simulink model "SST_v2_21b"  (R2021b)
settings: Solver=ode1be  StartTime=0.0  StopTime=1  FixedStep=Ts  RelTol=1e-3
values from neighbouring files (symbols this model uses):
  Kiv = 1/Tpv    (= 22527.3933103)    [DC_Grid_Light.m]
  Kpv = Tzv/Tpv    (= 0.187728277586)    [DC_Grid_Light.m]
undefined symbols (not defined in the file or in its folder): Cout, Imax, Kii, Kpi, Lfilter, Lgrid, Rfilter, Rgrid, RLoad, Ts, VAC_pk
libraries: simulink x62, spsVoltageMeasurementLib x21, spsParallelRLCBranchLib x15, spsFullBridgeConverterLib x15, spsACVoltageSourceLib x3, spsCurrentMeasurementLib x3, spsGroundLib x3, slpidlib x3, spsSeriesRLCBranchLib x3, spspowerguiLib x1
(part 1 of 2)
settings Model: Creator=velo  LastModifiedBy=MiguelVelo
settings DataIOCC: InitialState=out1.xFinal  SaveOperatingPoint=on
settings DebuggingCC: UnconnectedInputMsg=none  UnconnectedOutputMsg=none  UnconnectedLineMsg=none
settings ModelReferenceCC: EnableRefExpFcnMdlSchedulingChecks=off
settings RTWCC: GPUComputeCapability=5.0  DLArmComputeVersion=20.02.1

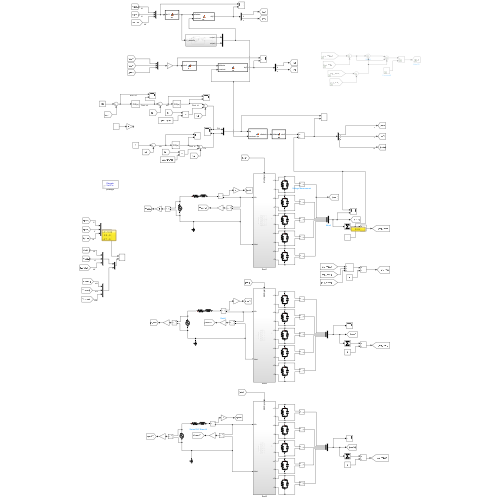
[thumbnail: Simulink's stored preview of the top-level diagram]
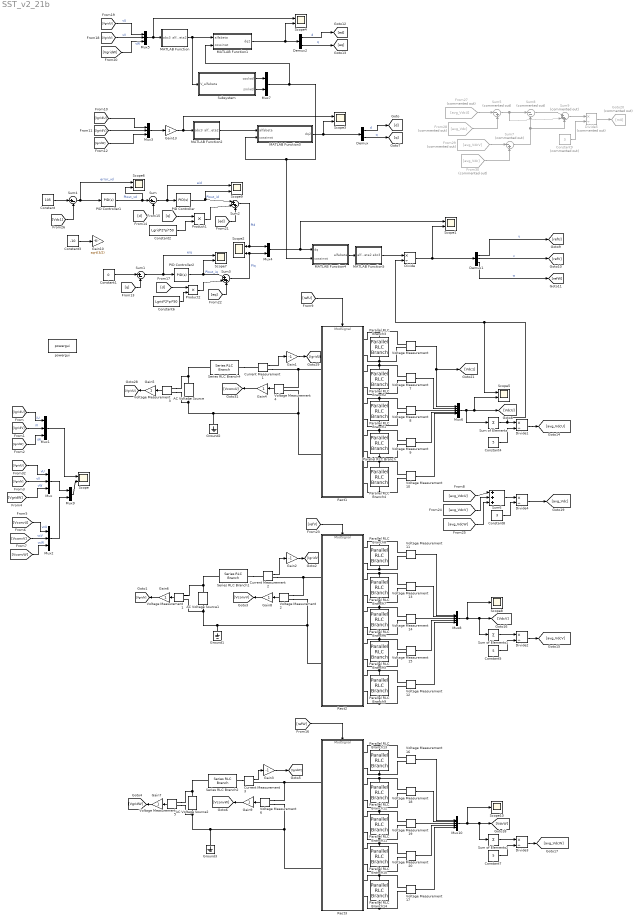
== system SST_v2_21b ==
  AC Voltage Source : spsACVoltageSourceLib/AC Voltage Source  Amplitude=VAC_pk  Phase=0  Frequency=50  SampleTime=0  Measurements=None  BusType=swing  Pref=10e3  Qref=0  Qmin=-inf  Qmax=+inf
  AC Voltage Source1 : spsACVoltageSourceLib/AC Voltage Source  Amplitude=VAC_pk  Phase=-120  Frequency=50  SampleTime=0  Measurements=None  BusType=swing  Pref=10e3  Qref=0  Qmin=-inf  Qmax=+inf
  AC Voltage Source2 : spsACVoltageSourceLib/AC Voltage Source  Amplitude=VAC_pk  Phase=120  Frequency=50  SampleTime=0  Measurements=None  BusType=swing  Pref=10e3  Qref=0  Qmin=-inf  Qmax=+inf
  Constant : Constant  Value=105
  Constant1 : Constant  Value=0
  Constant2 : Constant  Value=Lgrid*2*pi*50
  Constant3 : Constant  Value=-10
  Constant4 : Constant  Value=5
  Constant5 : Constant  Value=5
  Constant6 : Constant  Value=Lgrid*2*pi*50
  Constant7 : Constant  Value=5
  Constant8 : Constant  Value=3
  Constant9 : Constant  Commented=on  Value=3
  Current Measurement1 : spsCurrentMeasurementLib/Current Measurement  PhasorSimulation=off  OutputType=Complex  PSBequivalent=0
  Current Measurement2 : spsCurrentMeasurementLib/Current Measurement  PhasorSimulation=off  OutputType=Complex  PSBequivalent=0
  Current Measurement3 : spsCurrentMeasurementLib/Current Measurement  PhasorSimulation=off  OutputType=Complex  PSBequivalent=0
  Demux : Demux  Outputs=2
  Demux1 : Demux  Outputs=3
  Demux2 : Demux  Outputs=2
  Divide{,1..4} (5 alike) : Product  Inputs=*/
  Divide5 : Product  Commented=on  Inputs=*/
  From27 : From  Commented=on  GotoTag=avg_VdcU
  From28 : From  Commented=on  GotoTag=avg_Vdc
  From29 : From  Commented=on  GotoTag=avg_VdcV
  From30 : From  Commented=on  GotoTag=avg_Vdc
  Gain1 : Gain  Gain=-1
  Gain10 : Gain  Gain=sqrt(3/2)
  Gain{4..9,13} (7 alike) : Gain
  Gain2 : Gain  Gain=-1
  Gain3 : Gain  Gain=-1
  Goto20 : Goto  Commented=on  GotoTag=m0
  Ground1 : spsGroundLib/Ground  LConnTagsString=a
  Ground2 : spsGroundLib/Ground  LConnTagsString=a
  Ground3 : spsGroundLib/Ground  LConnTagsString=a
  MATLAB Function : MATLAB Function  TreatAsAtomicUnit=on
  MATLAB Function1 : MATLAB Function  TreatAsAtomicUnit=on
  MATLAB Function2 : MATLAB Function  TreatAsAtomicUnit=on
  MATLAB Function3 : MATLAB Function  TreatAsAtomicUnit=on
  MATLAB Function4 : MATLAB Function  TreatAsAtomicUnit=on
  MATLAB Function5 : MATLAB Function  TreatAsAtomicUnit=on
  Mux{,1..3,5} (5 alike) : Mux  Inputs=3
  Mux10 : Mux  Inputs=5
  Mux4 : Mux  Inputs=2
  Mux6 : Mux  Inputs=5
  Mux7 : Mux  Inputs=2
  Mux8 : Mux  Inputs=5
  Mux9 : Mux  Inputs=2
  PID Controller : slpidlib/PID Controller  Controller=PID  Form=Parallel  TimeDomain=Continuous-time  UseExternalTs=off  SampleTime=-1  IntegratorMethod=Forward Euler  FilterMethod=Forward Euler  ControllerParametersSource=internal  P=Kpi  I=Kii  D=0  UseFilter=on  N=100  TunerSelectOption=Transfer Function Based (PID Tuner App)  InitialConditionSource=internal  InitialConditionForIntegrator=0  InitialConditionForFilter=0  DifferentiatorICPrevScaledInput=0  ExternalReset=none  TrackingMode=off  Kt=1  LimitOutput=off  SatLimitsSource=internal  UpperSaturationLimit=Imax  LowerSaturationLimit=-Imax  LinearizeAsGain=on  AntiWindupMode=clamping  Kb=1  POutMin=[]  POutMax=[]  IOutMin=[]  IOutMax=[]  DOutMin=[]  DOutMax=[]  NOutMin=[]  NOutMax=[]  SumOutMin=[]  SumOutMax=[]  SaturationOutMin=[]  SaturationOutMax=[]  PParamMin=[]  PParamMax=[]  IParamMin=[]  IParamMax=[]  DParamMin=[]  DParamMax=[]  NParamMin=[]  NParamMax=[]  KbParamMin=[]  KbParamMax=[]  KtParamMin=[]  KtParamMax=[]  KbOutMin=[]  KbOutMax=[]  KtOutMin=[]  KtOutMax=[]  IntegratorOutMin=[]  IntegratorOutMax=[]  FilterOutMin=[]  FilterOutMax=[]  SumI1OutMin=[]  SumI1OutMax=[]  SumI2OutMin=[]  SumI2OutMax=[]  SumI3OutMin=[]  SumI3OutMax=[]  SumI4OutMin=[]  SumI4OutMax=[]  SumDOutMin=[]  SumDOutMax=[]  DifferentiatorOutMin=[]  DifferentiatorOutMax=[]  FilterDiffOutCoefMin=[]  FilterDiffOutCoefMax=[]  ReciprocalOutMin=[]  ReciprocalOutMax=[]  SumDenOutMin=[]  SumDenOutMax=[]  SumNumOutMin=[]  SumNumOutMax=[]  DivideOutMin=[]  DivideOutMax=[]  UdiffTsProdOutMin=[]  UdiffTsProdOutMax=[]  NTsProdOutMin=[]  NTsProdOutMax=[]  UintegralTsProdOutMin=[]  UintegralTsProdOutMax=[]  UngainTsProdOutMin=[]  UngainTsProdOutMax=[]  FilterDenConstantOutDataTypeStr=Inherit: Inherit via back propagation  FilterDenConstantOutMin=[]  FilterDenConstantOutMax=[]  PCopyOutDataTypeStr=Inherit: Inherit via back propagation  PCopyOutMin=[]  PCopyOutMax=[]  NCopyOutDataTypeStr=Inherit: Inherit via back propagation  NCopyOutMin=[]  NCopyOutMax=[]  IntegratorContinuousStateAttributes=''  IntegratorStateMustResolveToSignalObject=off  IntegratorRTWStateStorageClass=Auto  FilterContinuousStateAttributes=''  FilterStateMustResolveToSignalObject=off  FilterRTWStateStorageClass=Auto  ParallelPVariant=InternalParameters  IdealPVariant=Disabled  IVariant=InternalParameters  DVariant=InternalParameters  IntegratorVariant=Continuous  SatVariant=Disabled  AWVariant=Passthrough  PCopyVariant=Disabled  TRVariant=Disabled  FdbkBlocksVariant=Forward  IdealPFdbkVariant=Disabled  SatFdbkVariant=Disabled  DerivativeFilterVariant=ContFilter  NVariant=InternalParameters  NCopyVariant=Disabled  FilterICVariant=InternalICsFilter  IntegratorICVariant=InternalICs  ExternalResetVariant=Disabled  TRSumVariant=Passthrough  SumFdbkVariant=Disabled  SumVariant=Sum_PID  TsampFilterVariant=InternalTs  TsampNgainVariant=Passthrough  TsampIntegralVariant=Passthrough  ExternalSaturationOutDataTypeStr=Inherit: Same as second input
  PID Controller1 : slpidlib/PID Controller  Controller=PID  Form=Parallel  TimeDomain=Continuous-time  UseExternalTs=off  SampleTime=-1  IntegratorMethod=Forward Euler  FilterMethod=Forward Euler  ControllerParametersSource=internal  P=Kpv  I=Kiv  D=0  UseFilter=on  N=100  TunerSelectOption=Transfer Function Based (PID Tuner App)  InitialConditionSource=internal  InitialConditionForIntegrator=0  InitialConditionForFilter=0  DifferentiatorICPrevScaledInput=0  ExternalReset=none  TrackingMode=off  Kt=1  LimitOutput=off  SatLimitsSource=internal  UpperSaturationLimit=Imax  LowerSaturationLimit=-Imax  LinearizeAsGain=on  AntiWindupMode=clamping  Kb=1  POutMin=[]  POutMax=[]  IOutMin=[]  IOutMax=[]  DOutMin=[]  DOutMax=[]  NOutMin=[]  NOutMax=[]  SumOutMin=[]  SumOutMax=[]  SaturationOutMin=[]  SaturationOutMax=[]  PParamMin=[]  PParamMax=[]  IParamMin=[]  IParamMax=[]  DParamMin=[]  DParamMax=[]  NParamMin=[]  NParamMax=[]  KbParamMin=[]  KbParamMax=[]  KtParamMin=[]  KtParamMax=[]  KbOutMin=[]  KbOutMax=[]  KtOutMin=[]  KtOutMax=[]  IntegratorOutMin=[]  IntegratorOutMax=[]  FilterOutMin=[]  FilterOutMax=[]  SumI1OutMin=[]  SumI1OutMax=[]  SumI2OutMin=[]  SumI2OutMax=[]  SumI3OutMin=[]  SumI3OutMax=[]  SumI4OutMin=[]  SumI4OutMax=[]  SumDOutMin=[]  SumDOutMax=[]  DifferentiatorOutMin=[]  DifferentiatorOutMax=[]  FilterDiffOutCoefMin=[]  FilterDiffOutCoefMax=[]  ReciprocalOutMin=[]  ReciprocalOutMax=[]  SumDenOutMin=[]  SumDenOutMax=[]  SumNumOutMin=[]  SumNumOutMax=[]  DivideOutMin=[]  DivideOutMax=[]  UdiffTsProdOutMin=[]  UdiffTsProdOutMax=[]  NTsProdOutMin=[]  NTsProdOutMax=[]  UintegralTsProdOutMin=[]  UintegralTsProdOutMax=[]  UngainTsProdOutMin=[]  UngainTsProdOutMax=[]  FilterDenConstantOutDataTypeStr=Inherit: Inherit via back propagation  FilterDenConstantOutMin=[]  FilterDenConstantOutMax=[]  PCopyOutDataTypeStr=Inherit: Inherit via back propagation  PCopyOutMin=[]  PCopyOutMax=[]  NCopyOutDataTypeStr=Inherit: Inherit via back propagation  NCopyOutMin=[]  NCopyOutMax=[]  IntegratorContinuousStateAttributes=''  IntegratorStateMustResolveToSignalObject=off  IntegratorRTWStateStorageClass=Auto  FilterContinuousStateAttributes=''  FilterStateMustResolveToSignalObject=off  FilterRTWStateStorageClass=Auto  ParallelPVariant=InternalParameters  IdealPVariant=Disabled  IVariant=InternalParameters  DVariant=InternalParameters  IntegratorVariant=Continuous  SatVariant=Disabled  AWVariant=Passthrough  PCopyVariant=Disabled  TRVariant=Disabled  FdbkBlocksVariant=Forward  IdealPFdbkVariant=Disabled  SatFdbkVariant=Disabled  DerivativeFilterVariant=ContFilter  NVariant=InternalParameters  NCopyVariant=Disabled  FilterICVariant=InternalICsFilter  IntegratorICVariant=InternalICs  ExternalResetVariant=Disabled  TRSumVariant=Passthrough  SumFdbkVariant=Disabled  SumVariant=Sum_PID  TsampFilterVariant=InternalTs  TsampNgainVariant=Passthrough  TsampIntegralVariant=Passthrough  ExternalSaturationOutDataTypeStr=Inherit: Same as second input
  PID Controller2 : slpidlib/PID Controller  Controller=PID  Form=Parallel  TimeDomain=Continuous-time  UseExternalTs=off  SampleTime=-1  IntegratorMethod=Forward Euler  FilterMethod=Forward Euler  ControllerParametersSource=internal  P=Kpi  I=Kii  D=0  UseFilter=on  N=100  TunerSelectOption=Transfer Function Based (PID Tuner App)  InitialConditionSource=internal  InitialConditionForIntegrator=0  InitialConditionForFilter=0  DifferentiatorICPrevScaledInput=0  ExternalReset=none  TrackingMode=off  Kt=1  LimitOutput=off  SatLimitsSource=internal  UpperSaturationLimit=Imax  LowerSaturationLimit=-Imax  LinearizeAsGain=on  AntiWindupMode=clamping  Kb=1  POutMin=[]  POutMax=[]  IOutMin=[]  IOutMax=[]  DOutMin=[]  DOutMax=[]  NOutMin=[]  NOutMax=[]  SumOutMin=[]  SumOutMax=[]  SaturationOutMin=[]  SaturationOutMax=[]  PParamMin=[]  PParamMax=[]  IParamMin=[]  IParamMax=[]  DParamMin=[]  DParamMax=[]  NParamMin=[]  NParamMax=[]  KbParamMin=[]  KbParamMax=[]  KtParamMin=[]  KtParamMax=[]  KbOutMin=[]  KbOutMax=[]  KtOutMin=[]  KtOutMax=[]  IntegratorOutMin=[]  IntegratorOutMax=[]  FilterOutMin=[]  FilterOutMax=[]  SumI1OutMin=[]  SumI1OutMax=[]  SumI2OutMin=[]  SumI2OutMax=[]  SumI3OutMin=[]  SumI3OutMax=[]  SumI4OutMin=[]  SumI4OutMax=[]  SumDOutMin=[]  SumDOutMax=[]  DifferentiatorOutMin=[]  DifferentiatorOutMax=[]  FilterDiffOutCoefMin=[]  FilterDiffOutCoefMax=[]  ReciprocalOutMin=[]  ReciprocalOutMax=[]  SumDenOutMin=[]  SumDenOutMax=[]  SumNumOutMin=[]  SumNumOutMax=[]  DivideOutMin=[]  DivideOutMax=[]  UdiffTsProdOutMin=[]  UdiffTsProdOutMax=[]  NTsProdOutMin=[]  NTsProdOutMax=[]  UintegralTsProdOutMin=[]  UintegralTsProdOutMax=[]  UngainTsProdOutMin=[]  UngainTsProdOutMax=[]  FilterDenConstantOutDataTypeStr=Inherit: Inherit via back propagation  FilterDenConstantOutMin=[]  FilterDenConstantOutMax=[]  PCopyOutDataTypeStr=Inherit: Inherit via back propagation  PCopyOutMin=[]  PCopyOutMax=[]  NCopyOutDataTypeStr=Inherit: Inherit via back propagation  NCopyOutMin=[]  NCopyOutMax=[]  IntegratorContinuousStateAttributes=''  IntegratorStateMustResolveToSignalObject=off  IntegratorRTWStateStorageClass=Auto  FilterContinuousStateAttributes=''  FilterStateMustResolveToSignalObject=off  FilterRTWStateStorageClass=Auto  ParallelPVariant=InternalParameters  IdealPVariant=Disabled  IVariant=InternalParameters  DVariant=InternalParameters  IntegratorVariant=Continuous  SatVariant=Disabled  AWVariant=Passthrough  PCopyVariant=Disabled  TRVariant=Disabled  FdbkBlocksVariant=Forward  IdealPFdbkVariant=Disabled  SatFdbkVariant=Disabled  DerivativeFilterVariant=ContFilter  NVariant=InternalParameters  NCopyVariant=Disabled  FilterICVariant=InternalICsFilter  IntegratorICVariant=InternalICs  ExternalResetVariant=Disabled  TRSumVariant=Passthrough  SumFdbkVariant=Disabled  SumVariant=Sum_PID  TsampFilterVariant=InternalTs  TsampNgainVariant=Passthrough  TsampIntegralVariant=Passthrough  ExternalSaturationOutDataTypeStr=Inherit: Same as second input
  Parallel RLC Branch{,1..14} (15 alike) : spsParallelRLCBranchLib/Parallel RLC Branch  LConnTagsString=a  RConnTagsString=__new0  BranchType=RC  Resistance=RLoad  Inductance=1e-3  SetiL0=off  InitialCurrent=0  Capacitance=Cout  Setx0=on  InitialVoltage=Initial_Cap_V  Measurements=None
  Product1 : Product
  Product2 : Product
  Rect1 : Subsystem
      settings: PortSchema="{\"entries\":[{\"content\":{\"sides\":[{\"content\":{\"connectorIds\":[\"LConn1\",\"LConn2\"]},\"type\":\"ConnectorPlacement.EquallySpacedRectSide\",\"uuid\":\"6da19801-630c-4f3f-87cc-390789255ba0\"},{\"content\":{\"connectorIds\":[\"RConn1\",\"RConn2\",\"RConn3\",\"RConn4\",\"RConn5\",\"RConn6\",\"RConn7\",\"RConn8\",\"RConn9\",\"RConn10\"],\"side\":\"RIGHT\"},\"type\":\"ConnectorPlacement.EquallySpacedRectSide\",\"uuid\":\"ec1a5a2a-530e-42f7-98ba-80a24dcc9532\"},{\"content\":{\"connectorIds\":[\"In1\"],\"side\":\"TOP\"},\"type\":\"ConnectorPlacement.EquallySpacedRectSide\",\"uuid\":\"a1ee5919-0a6c-4c11-9fd8-b0a64dbbf7b8\"}]},\"type\":\"ConnectorPlacement.EquallySpacedConnector\",\"uuid\":\"d117ce62-6661-4f44-89fc-3a19d4e0e3a2\"}],\"packageUris\":[\"http://schema.mathworks.com/mf0/Connector/R2020b\"],\"version\":\"1.0\"}"
  Rect2 : Subsystem
      settings: PortSchema="{\"entries\":[{\"content\":{\"sides\":[{\"content\":{\"connectorIds\":[\"LConn1\",\"LConn2\"]},\"type\":\"ConnectorPlacement.EquallySpacedRectSide\",\"uuid\":\"6da19801-630c-4f3f-87cc-390789255ba0\"},{\"content\":{\"connectorIds\":[\"RConn1\",\"RConn2\",\"RConn3\",\"RConn4\",\"RConn5\",\"RConn6\",\"RConn7\",\"RConn8\",\"RConn9\",\"RConn10\"],\"side\":\"RIGHT\"},\"type\":\"ConnectorPlacement.EquallySpacedRectSide\",\"uuid\":\"ec1a5a2a-530e-42f7-98ba-80a24dcc9532\"},{\"content\":{\"connectorIds\":[\"In1\"],\"side\":\"TOP\"},\"type\":\"ConnectorPlacement.EquallySpacedRectSide\",\"uuid\":\"a1ee5919-0a6c-4c11-9fd8-b0a64dbbf7b8\"}]},\"type\":\"ConnectorPlacement.EquallySpacedConnector\",\"uuid\":\"d117ce62-6661-4f44-89fc-3a19d4e0e3a2\"}],\"packageUris\":[\"http://schema.mathworks.com/mf0/Connector/R2020b\"],\"version\":\"1.0\"}"
  Rect3 : Subsystem
      settings: PortSchema="{\"entries\":[{\"content\":{\"sides\":[{\"content\":{\"connectorIds\":[\"LConn1\",\"LConn2\"]},\"type\":\"ConnectorPlacement.EquallySpacedRectSide\",\"uuid\":\"6da19801-630c-4f3f-87cc-390789255ba0\"},{\"content\":{\"connectorIds\":[\"RConn1\",\"RConn2\",\"RConn3\",\"RConn4\",\"RConn5\",\"RConn6\",\"RConn7\",\"RConn8\",\"RConn9\",\"RConn10\"],\"side\":\"RIGHT\"},\"type\":\"ConnectorPlacement.EquallySpacedRectSide\",\"uuid\":\"ec1a5a2a-530e-42f7-98ba-80a24dcc9532\"},{\"content\":{\"connectorIds\":[\"In1\"],\"side\":\"TOP\"},\"type\":\"ConnectorPlacement.EquallySpacedRectSide\",\"uuid\":\"a1ee5919-0a6c-4c11-9fd8-b0a64dbbf7b8\"}]},\"type\":\"ConnectorPlacement.EquallySpacedConnector\",\"uuid\":\"d117ce62-6661-4f44-89fc-3a19d4e0e3a2\"}],\"packageUris\":[\"http://schema.mathworks.com/mf0/Connector/R2020b\"],\"version\":\"1.0\"}"
  Scope{,1..7,9} (9 alike) : Scope  NumInputPorts=2
  Scope10 : Scope
  Scope8 : Scope
  Series RLC Branch1 : spsSeriesRLCBranchLib/Series RLC Branch  LConnTagsString=__new0  RConnTagsString=__new0  BranchType=RL  Resistance=Rfilter+Rgrid  Inductance=Lfilter+Lgrid  SetiL0=off  InitialCurrent=0  Capacitance=1e-6  Setx0=off  InitialVoltage=0  Measurements=None
  Series RLC Branch2 : spsSeriesRLCBranchLib/Series RLC Branch  LConnTagsString=__new0  RConnTagsString=__new0  BranchType=RL  Resistance=Rfilter+Rgrid  Inductance=Lfilter+Lgrid  SetiL0=off  InitialCurrent=0  Capacitance=1e-6  Setx0=off  InitialVoltage=0  Measurements=None
  Series RLC Branch4 : spsSeriesRLCBranchLib/Series RLC Branch  LConnTagsString=__new0  RConnTagsString=__new0  BranchType=RL  Resistance=Rfilter+Rgrid  Inductance=Lfilter+Lgrid  SetiL0=off  InitialCurrent=0  Capacitance=1e-6  Setx0=off  InitialVoltage=0  Measurements=None
  Subsystem : Subsystem
  Sum : Sum  Inputs=|+-
  Sum of Elements : Sum  Inputs=+
  Sum of Elements1 : Sum  Inputs=+
  Sum of Elements2 : Sum  Inputs=+
  Sum1 : Sum  Inputs=|+-
  Sum2 : Sum  Inputs=|+-+
  Sum3 : Sum  Inputs=|+++
  Sum4 : Sum  Inputs=|+-
  Sum5 : Sum  Commented=on  Inputs=|-+
  Sum6 : Sum  Inputs=|+++
  Sum7 : Sum  Commented=on  Inputs=|-+
  Sum8 : Sum  Commented=on  Inputs=|--
  Sum9 : Sum  Commented=on  Inputs=|+++
  Voltage Measurement{,1..20} (21 alike) : spsVoltageMeasurementLib/Voltage Measurement  PhasorSimulation=off  OutputType=Complex  PSBequivalent=0
  powergui : spspowerguiLib/powergui  Priority=1  SimulationMode=Discrete  SampleTime=Ts  frequency=60  Iterations=50  frequencyindice=0  Pbase=100e6  ErrMax=1e-4  UnitsV=kV  UnitsW=MW  buscounter=0  FunctionMessages=off  echomessages=off  EnableUseOfTLC=off  CurrentSourceSwitches=off  DisableSnubberDevices=off  DisableRonSwitches=off  DisableVfSwitches=off  DisplayEquations=off  AutomaticDiscreteSolvers=on  SolverType=Tustin/Backward Euler (TBE)  Interpol=off  ExternalGateDelay=off  methode=off  Ts=100  x0status=blocks  SPID=on  SwTol=0  HookPort=off  NonlinearTolerance=1e-4  nMaxIteration=100  ContinueOnMaxIteration=off  RestoreLinks=warning  ResistiveCurrentMeasurement=off  Frange=[0:2:500]  Ylog=off  Xlog=on  ShowGrid=off  save=off  variable=ZData  structure=0  ZoomFFT=off  StartTime=0.0  cycles=1  DisplayStyle=1  fundamental=60  FreqAxis=off  MaxFrequency=1000  frequencyindicesteady=1  RmsSteady=1  display=off
  wires:
  [VgridU] -> Mux/1  "vU"
  Voltage Measurement3/1 -> Gain5/1
  Current Measurement1/1 -> Gain1/1
  Gain4/1 -> [VconvU]
  Voltage Measurement2/1 -> Gain8/1
  Current Measurement2/1 -> Gain2/1
  Current Measurement3/1 -> Gain3/1
  Voltage Measurement6/1 -> Gain9/1
  [IgridU] -> Mux1/1  "iU"
  [IgridV] -> Mux1/2  "iV"
  [IgridW] -> Mux1/3  "iW"
  Mux1/1 -> Scope/1
  [VgridV] -> Mux/2  "vV"
  [VgridW] -> Mux/3  "vW"
  Mux/1 -> Mux9/1
  [VconvU] -> Mux2/1  "vcU"
  [VconvV] -> Mux2/2  "vcV"
  [VconvW] -> Mux2/3  "vcW"
  Mux2/1 -> Mux9/2
  Mux3/1 -> Gain13/1
  Demux/1 -> [d]  "d"
  Demux/2 -> [q]  "q"
  [d] -> Sum/2
  Constant1/1 -> Sum1/1
  Sum2/1 -> Mux4/1, Scope2/1  "PId"
  MATLAB Function1/1(dq2) -> Demux2/1, Scope4/2
  Sum3/1 -> Mux4/2, Scope2/2  "PIq"
  PID Controller2/1 -> Scope7/2, Sum3/1  "PIout_iq"
  [q] -> Sum1/2
  Product1/1 -> Sum2/2
  [q] -> Product1/1
  Product2/1 -> Sum3/2
  [d] -> Product2/1
  [IgridU] -> Mux3/1
  [IgridV] -> Mux3/2
  [IgridW] -> Mux3/3
  PID Controller/1 -> Scope9/2, Sum2/1  "PIout_id"
  Constant2/1 -> Product1/2
  Constant6/1 -> Product2/2
  Demux2/1 -> [ed]  "d"
  Demux2/2 -> [eq]  "q"
  MATLAB Function5/1(abc3) -> Divide/1
  Gain1/1 -> [IgridU]
  Gain2/1 -> [IgridV]
  Gain3/1 -> [IgridW]
  Sum/1 -> Scope9/1, PID Controller/1  "eid"
  Sum1/1 -> Scope7/1, PID Controller2/1  "eiq"
  Divide/1 -> Scope1/2, Demux1/1
  [ed] -> Sum2/3
  [eq] -> Sum3/3
  Gain5/1 -> [VgridU]
  Gain6/1 -> [VgridV]
  Voltage Measurement1/1 -> Gain6/1
  Gain7/1 -> [VgridW]
  Voltage Measurement5/1 -> Gain7/1
  Voltage Measurement4/1 -> Gain4/1
  Gain8/1 -> [VconvV]
  Gain9/1 -> [VconvW]
  [refU] -> Rect1/1(ModSignal)
  [refV] -> Rect2/1(ModSignal)
  [refW] -> Rect3/1(ModSignal)
  Mux5/1 -> Scope4/1, MATLAB Function/1(abc3)
  Gain13/1 -> Scope3/1, MATLAB Function2/1(abc3)
  MATLAB Function/1(alfabeta2) -> Subsystem/1(V_alfabeta), MATLAB Function1/1(alfabeta)
  Subsystem/1(cos(wt)) -> Mux7/1
  Subsystem/2(sin(wt)) -> Mux7/2
  MATLAB Function2/1(alfabeta2) -> MATLAB Function3/1(alfabeta)
  Mux7/1 -> MATLAB Function1/2(cossinwt), MATLAB Function3/2(cossinwt), MATLAB Function4/2(cossinwt)
  MATLAB Function3/1(dq2) -> Demux/1, Scope3/2
  MATLAB Function4/1(alfabeta) -> MATLAB Function5/1(alfabeta2)
  Mux9/1 -> Scope/2
  Mux4/1 -> Scope1/1, MATLAB Function4/1(dq)
  [VgridV] -> Mux5/2  "vV"
  [VgridW] -> Mux5/3  "vW"
  [VgridU] -> Mux5/1  "vU"
  Constant/1 -> Sum4/1
  Sum4/1 -> Scope6/1, PID Controller1/1  "error_vd"
  [Vdc1] -> Sum4/2
  Voltage Measurement/1 -> [Vdc1], Mux6/1
  Voltage Measurement7/1 -> Mux6/2
  Voltage Measurement8/1 -> Mux6/3
  Voltage Measurement9/1 -> Mux6/4
  Voltage Measurement10/1 -> Mux6/5
  Mux6/1 -> Sum of Elements/1, [VdcU], Scope5/2
  Constant3/1 -> Gain10/1
  PID Controller1/1 -> Scope6/2, Sum/1  "PIout_vd"
  Voltage Measurement15/1 -> Mux8/4
  Voltage Measurement12/1 -> Mux8/5
  Voltage Measurement14/1 -> Mux8/3
  Voltage Measurement13/1 -> Mux8/2
  Voltage Measurement11/1 -> Mux8/1
  Voltage Measurement20/1 -> Mux10/4
  Voltage Measurement16/1 -> Mux10/1
  Voltage Measurement17/1 -> Mux10/5
  Voltage Measurement19/1 -> Mux10/3
  Voltage Measurement18/1 -> Mux10/2
  Constant4/1 -> Divide1/2
  Divide1/1 -> [avg_VdcU]
  Mux8/1 -> Sum of Elements1/1, [VdcV], Scope8/1
  Constant5/1 -> Divide2/2
  Sum of Elements1/1 -> Divide2/1
  Divide2/1 -> [avg_VdcV]
  Constant7/1 -> Divide3/2
  Sum of Elements2/1 -> Divide3/1
  Divide3/1 -> [avg_VdcW]
  Mux10/1 -> Sum of Elements2/1, [VdcW], Scope10/1
  [avg_VdcU] -> Sum6/1
  [avg_VdcV] -> Sum6/2
  [avg_VdcW] -> Sum6/3
  Sum6/1 -> Divide4/1
  Constant8/1 -> Divide4/2
  Divide4/1 -> [avg_Vdc]
  From27/1 -> Sum5/1
  From28/1 -> Sum5/2
  From30/1 -> Sum7/2
  From29/1 -> Sum7/1
  Sum5/1 -> Sum9/2, Sum8/1
  Sum7/1 -> Sum9/3, Sum8/2
  Sum8/1 -> Sum9/1
  Sum9/1 -> Divide5/1
  Constant9/1 -> Divide5/2
  Divide5/1 -> Goto20/1
  Demux1/1 -> [refU]  "u"
  Demux1/2 -> [refV]  "v"
  Demux1/3 -> [refW]  "w"
  Sum of Elements/1 -> Scope5/1, Divide/2, Divide1/1
  connections:
  Series RLC Branch4/RConn1 -- Current Measurement1/LConn1
  Voltage Measurement2/LConn1 -- Rect2/LConn1 -- Current Measurement2/RConn1
  Series RLC Branch1/RConn1 -- Current Measurement2/LConn1
  Voltage Measurement6/LConn1 -- Rect3/LConn1 -- Current Measurement3/RConn1
  AC Voltage Source2/RConn1 -- Series RLC Branch2/LConn1 -- Voltage Measurement5/LConn1
  Series RLC Branch2/RConn1 -- Current Measurement3/LConn1
  Parallel RLC Branch/RConn1 -- Rect1/RConn8 -- Voltage Measurement9/LConn2
  Parallel RLC Branch/LConn1 -- Rect1/RConn7 -- Voltage Measurement9/LConn1
  Parallel RLC Branch1/LConn1 -- Rect1/RConn5 -- Voltage Measurement8/LConn1
  Rect1/RConn6 -- Voltage Measurement8/LConn2 -- Parallel RLC Branch1/RConn1
  Parallel RLC Branch2/RConn1 -- Voltage Measurement7/LConn2 -- Rect1/RConn4
  Parallel RLC Branch2/LConn1 -- Voltage Measurement7/LConn1 -- Rect1/RConn3
  Parallel RLC Branch3/LConn1 -- Rect1/RConn1 -- Voltage Measurement/LConn1
  Parallel RLC Branch3/RConn1 -- Voltage Measurement/LConn2 -- Rect1/RConn2
  Parallel RLC Branch4/LConn1 -- Rect1/RConn9 -- Voltage Measurement10/LConn1
  Parallel RLC Branch4/RConn1 -- Rect1/RConn10 -- Voltage Measurement10/LConn2
  Parallel RLC Branch9/RConn1 -- Rect2/RConn10 -- Voltage Measurement12/LConn2
  Parallel RLC Branch6/LConn1 -- Rect2/RConn5 -- Voltage Measurement14/LConn1
  Parallel RLC Branch5/RConn1 -- Rect2/RConn8 -- Voltage Measurement15/LConn2
  Parallel RLC Branch7/LConn1 -- Rect2/RConn3 -- Voltage Measurement13/LConn1
  Parallel RLC Branch8/LConn1 -- Rect2/RConn1 -- Voltage Measurement11/LConn1
  Parallel RLC Branch5/LConn1 -- Rect2/RConn7 -- Voltage Measurement15/LConn1
  Parallel RLC Branch8/RConn1 -- Rect2/RConn2 -- Voltage Measurement11/LConn2
  Parallel RLC Branch7/RConn1 -- Rect2/RConn4 -- Voltage Measurement13/LConn2
  Parallel RLC Branch9/LConn1 -- Rect2/RConn9 -- Voltage Measurement12/LConn1
  Parallel RLC Branch6/RConn1 -- Rect2/RConn6 -- Voltage Measurement14/LConn2
  Parallel RLC Branch14/RConn1 -- Rect3/RConn10 -- Voltage Measurement17/LConn2
  Parallel RLC Branch11/LConn1 -- Rect3/RConn5 -- Voltage Measurement19/LConn1
  Parallel RLC Branch11/RConn1 -- Rect3/RConn6 -- Voltage Measurement19/LConn2
  Parallel RLC Branch12/LConn1 -- Rect3/RConn3 -- Voltage Measurement18/LConn1
  Parallel RLC Branch10/RConn1 -- Rect3/RConn8 -- Voltage Measurement20/LConn2
  Parallel RLC Branch13/LConn1 -- Rect3/RConn1 -- Voltage Measurement16/LConn1
  Parallel RLC Branch10/LConn1 -- Rect3/RConn7 -- Voltage Measurement20/LConn1
  Parallel RLC Branch14/LConn1 -- Rect3/RConn9 -- Voltage Measurement17/LConn1
  Parallel RLC Branch13/RConn1 -- Rect3/RConn2 -- Voltage Measurement16/LConn2
  Parallel RLC Branch12/RConn1 -- Rect3/RConn4 -- Voltage Measurement18/LConn2
  Rect1/LConn1 -- Current Measurement1/RConn1 -- Voltage Measurement4/LConn1
  Voltage Measurement6/LConn2 -- Rect3/LConn2 -- Voltage Measurement5/LConn2 -- AC Voltage Source2/LConn1 -- Ground3/LConn1
  Voltage Measurement3/LConn1 -- Series RLC Branch4/LConn1 -- AC Voltage Source/RConn1
  Voltage Measurement3/LConn2 -- Ground2/LConn1 -- Rect1/LConn2 -- Voltage Measurement4/LConn2 -- AC Voltage Source/LConn1
  Voltage Measurement2/LConn2 -- Rect2/LConn2 -- AC Voltage Source1/LConn1 -- Voltage Measurement1/LConn2 -- Ground1/LConn1
  Voltage Measurement1/LConn1 -- Series RLC Branch1/LConn1 -- AC Voltage Source1/RConn1

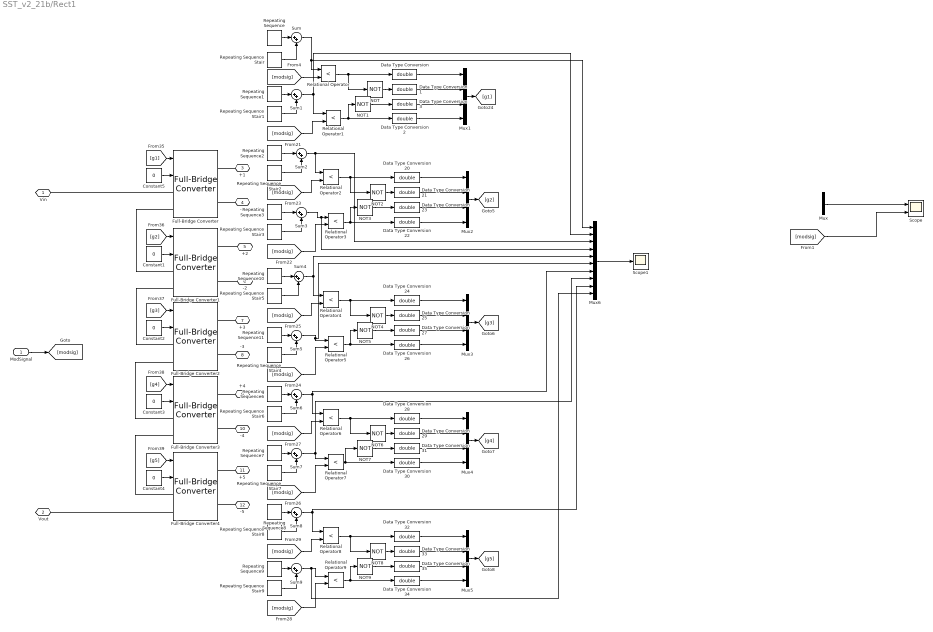
== system SST_v2_21b/Rect1 ==
  ModSignal : Inport
  Constant{1..5} (5 alike) : Constant  Value=0
  Data Type Conversion{,1..3,20..35} (20 alike) : DataTypeConversion  OutMin=[0]  OutMax=[1]  OutDataTypeStr=double
  Full-Bridge Converter{,1..4} (5 alike) : spsFullBridgeConverterLib/Full-Bridge Converter  ModelType=Switching devices  Ron=Rdson  Rs=Rsnubber  Cs=Csnubber  Vforward=[0,0]  Ron_Diode=1e-3  Rs_Diode=1e6  Cs_Diode=inf  Vf_Diode=1e-3  Rs_CurrentSource=inf
      settings: SourceProductBaseCode=PS
  Mux : Mux  Inputs=10
  Mux{1..5} (5 alike) : Mux
  Mux6 : Mux  Inputs=10
  NOT{,1..9} (10 alike) : Logic  Operator=NOT  IconShape=distinctive  AllPortsSameDT=off  OutDataTypeStr=boolean
  Relational Operator{,1..9} (10 alike) : RelationalOperator  Operator=<  OutDataTypeStr=boolean  RndMeth=Simplest
  Repeating Sequence : simulink/Sources/Repeating Sequence  rep_seq_t=Tcarriers  rep_seq_y=Ac11
  Repeating Sequence Stair : simulink/Sources/Repeating Sequence Stair  OutValues=Sc11  tsamp=TswS  OutMin=[]  OutMax=[]  OutDataTypeStr=double  OutputDataTypeScalingMode=double  OutDataType=fixdt(0,8)  ConRadixGroup=Best Precision: Vector-wise  OutScaling=2^-12
  Repeating Sequence Stair1 : simulink/Sources/Repeating Sequence Stair  OutValues=Sc12  tsamp=TswS  OutMin=[]  OutMax=[]  OutDataTypeStr=double  OutputDataTypeScalingMode=double  OutDataType=fixdt(0,8)  ConRadixGroup=Best Precision: Vector-wise  OutScaling=2^-12
  Repeating Sequence Stair2 : simulink/Sources/Repeating Sequence Stair  OutValues=Sc21  tsamp=TswS  OutMin=[]  OutMax=[]  OutDataTypeStr=double  OutputDataTypeScalingMode=double  OutDataType=fixdt(0,8)  ConRadixGroup=Best Precision: Vector-wise  OutScaling=2^-12
  Repeating Sequence Stair3 : simulink/Sources/Repeating Sequence Stair  OutValues=Sc22  tsamp=TswS  OutMin=[]  OutMax=[]  OutDataTypeStr=double  OutputDataTypeScalingMode=double  OutDataType=fixdt(0,8)  ConRadixGroup=Best Precision: Vector-wise  OutScaling=2^-12
  Repeating Sequence Stair4 : simulink/Sources/Repeating Sequence Stair  OutValues=Sc32  tsamp=TswS  OutMin=[]  OutMax=[]  OutDataTypeStr=double  OutputDataTypeScalingMode=double  OutDataType=fixdt(0,8)  ConRadixGroup=Best Precision: Vector-wise  OutScaling=2^-12
  Repeating Sequence Stair5 : simulink/Sources/Repeating Sequence Stair  OutValues=Sc31  tsamp=TswS  OutMin=[]  OutMax=[]  OutDataTypeStr=double  OutputDataTypeScalingMode=double  OutDataType=fixdt(0,8)  ConRadixGroup=Best Precision: Vector-wise  OutScaling=2^-12
  Repeating Sequence Stair6 : simulink/Sources/Repeating Sequence Stair  OutValues=Sc41  tsamp=TswS  OutMin=[]  OutMax=[]  OutDataTypeStr=double  OutputDataTypeScalingMode=double  OutDataType=fixdt(0,8)  ConRadixGroup=Best Precision: Vector-wise  OutScaling=2^-12
  Repeating Sequence Stair7 : simulink/Sources/Repeating Sequence Stair  OutValues=Sc42  tsamp=TswS  OutMin=[]  OutMax=[]  OutDataTypeStr=double  OutputDataTypeScalingMode=double  OutDataType=fixdt(0,8)  ConRadixGroup=Best Precision: Vector-wise  OutScaling=2^-12
  Repeating Sequence Stair8 : simulink/Sources/Repeating Sequence Stair  OutValues=Sc51  tsamp=TswS  OutMin=[]  OutMax=[]  OutDataTypeStr=double  OutputDataTypeScalingMode=double  OutDataType=fixdt(0,8)  ConRadixGroup=Best Precision: Vector-wise  OutScaling=2^-12
  Repeating Sequence Stair9 : simulink/Sources/Repeating Sequence Stair  OutValues=Sc52  tsamp=TswS  OutMin=[]  OutMax=[]  OutDataTypeStr=double  OutputDataTypeScalingMode=double  OutDataType=fixdt(0,8)  ConRadixGroup=Best Precision: Vector-wise  OutScaling=2^-12
  Repeating Sequence1 : simulink/Sources/Repeating Sequence  rep_seq_t=Tcarriers  rep_seq_y=AC12
  Repeating Sequence10 : simulink/Sources/Repeating Sequence  rep_seq_t=Tcarriers  rep_seq_y=Ac31
  Repeating Sequence11 : simulink/Sources/Repeating Sequence  rep_seq_t=Tcarriers  rep_seq_y=AC32
  Repeating Sequence2 : simulink/Sources/Repeating Sequence  rep_seq_t=Tcarriers  rep_seq_y=Ac21
  Repeating Sequence3 : simulink/Sources/Repeating Sequence  rep_seq_t=Tcarriers  rep_seq_y=Ac22
  Repeating Sequence6 : simulink/Sources/Repeating Sequence  rep_seq_t=Tcarriers  rep_seq_y=Ac41
  Repeating Sequence7 : simulink/Sources/Repeating Sequence  rep_seq_t=Tcarriers  rep_seq_y=Ac42
  Repeating Sequence8 : simulink/Sources/Repeating Sequence  rep_seq_t=Tcarriers  rep_seq_y=Ac51
  Repeating Sequence9 : simulink/Sources/Repeating Sequence  rep_seq_t=Tcarriers  rep_seq_y=Ac52
  Scope : Scope  NumInputPorts=2
  Scope1 : Scope
  Sum{,1..9} (10 alike) : Sum  Inputs=|++
  Vin : PMIOPort  Side=Left
  Vout : PMIOPort  Port=2  Side=Left
  +1 : PMIOPort  Port=3  Side=Right
  -1 : PMIOPort  Port=4  Side=Right
  +2 : PMIOPort  Port=5  Side=Right
  -2 : PMIOPort  Port=6  Side=Right
  +3 : PMIOPort  Port=7  Side=Right
  -3 : PMIOPort  Port=8  Side=Right
  +4 : PMIOPort  Port=9  Side=Right
  -4 : PMIOPort  Port=10  Side=Right
  +5 : PMIOPort  Port=11  Side=Right
  -5 : PMIOPort  Port=12  Side=Right
  wires:
  Data Type Conversion/1 -> Mux1/1
  [modsig] -> Relational Operator7/2
  Data Type Conversion33/1 -> Mux5/2
  NOT2/1 -> Data Type Conversion21/1
  Data Type Conversion30/1 -> Mux4/4
  Constant5/1 -> Full-Bridge Converter/2
  Data Type Conversion31/1 -> Mux4/3
  Data Type Conversion23/1 -> Mux2/3
  [g4] -> Full-Bridge Converter3/1
  NOT8/1 -> Data Type Conversion33/1
  Constant4/1 -> Full-Bridge Converter4/2
  Data Type Conversion29/1 -> Mux4/2
  Data Type Conversion24/1 -> Mux3/1
  Data Type Conversion25/1 -> Mux3/2
  NOT7/1 -> Data Type Conversion31/1
  Mux5/1 -> [g5]
  [g1] -> Full-Bridge Converter/1
  NOT5/1 -> Data Type Conversion27/1
  NOT3/1 -> Data Type Conversion23/1
  Relational Operator8/1 -> Data Type Conversion32/1, NOT8/1
  Data Type Conversion26/1 -> Mux3/4
  [modsig] -> Relational Operator6/2
  Relational Operator3/1 -> Data Type Conversion22/1, NOT3/1
  Mux1/1 -> [g1]
  Constant2/1 -> Full-Bridge Converter2/2
  Data Type Conversion3/1 -> Mux1/3
  Mux4/1 -> [g4]
  Relational Operator5/1 -> Data Type Conversion26/1, NOT5/1
  Relational Operator1/1 -> Data Type Conversion2/1, NOT1/1
  Constant1/1 -> Full-Bridge Converter1/2
  [modsig] -> Relational Operator3/2
  Relational Operator/1 -> Data Type Conversion/1, NOT/1
  [g2] -> Full-Bridge Converter1/1
  Mux2/1 -> [g2]
  Relational Operator4/1 -> Data Type Conversion24/1, NOT4/1
  [modsig] -> Relational Operator/2
  [modsig] -> Relational Operator9/2
  Data Type Conversion32/1 -> Mux5/1
  NOT/1 -> Data Type Conversion1/1
  Data Type Conversion35/1 -> Mux5/3
  Relational Operator6/1 -> Data Type Conversion28/1, NOT6/1
  [modsig] -> Relational Operator1/2
  NOT6/1 -> Data Type Conversion29/1
  NOT1/1 -> Data Type Conversion3/1
  [modsig] -> Relational Operator5/2
  Data Type Conversion21/1 -> Mux2/2
  Data Type Conversion27/1 -> Mux3/3
  Relational Operator2/1 -> Data Type Conversion20/1, NOT2/1
  Mux3/1 -> [g3]
  Relational Operator7/1 -> Data Type Conversion30/1, NOT7/1
  Data Type Conversion34/1 -> Mux5/4
  [modsig] -> Relational Operator4/2
  NOT9/1 -> Data Type Conversion35/1
  [g3] -> Full-Bridge Converter2/1
  Data Type Conversion28/1 -> Mux4/1
  Data Type Conversion20/1 -> Mux2/1
  Repeating Sequence3/1 -> Sum3/1
  [modsig] -> Relational Operator2/2
  Relational Operator9/1 -> Data Type Conversion34/1, NOT9/1
  [modsig] -> Relational Operator8/2
  Constant3/1 -> Full-Bridge Converter3/2
  Data Type Conversion1/1 -> Mux1/2
  NOT4/1 -> Data Type Conversion25/1
  Data Type Conversion2/1 -> Mux1/4
  Data Type Conversion22/1 -> Mux2/4
  [g5] -> Full-Bridge Converter4/1
  ModSignal/1 -> [modsig]
  Mux/1 -> Scope/1
  [modsig] -> Scope/2
  Repeating Sequence/1 -> Sum/1
  Sum/1 -> Mux6/1, Relational Operator/1
  Repeating Sequence1/1 -> Sum1/1
  Repeating Sequence Stair1/1 -> Sum1/2
  Sum1/1 -> Relational Operator1/1, Mux6/2
  Repeating Sequence2/1 -> Sum2/1
  Repeating Sequence Stair2/1 -> Sum2/2
  Sum2/1 -> Mux6/3, Relational Operator2/1
  Sum3/1 -> Mux6/4, Relational Operator3/1
  Repeating Sequence Stair3/1 -> Sum3/2
  Repeating Sequence10/1 -> Sum4/1
  Repeating Sequence Stair5/1 -> Sum4/2
  Sum4/1 -> Relational Operator4/1, Mux6/5
  Repeating Sequence11/1 -> Sum5/1
  Sum5/1 -> Mux6/6, Relational Operator5/1
  Repeating Sequence Stair4/1 -> Sum5/2
  Repeating Sequence6/1 -> Sum6/1
  Repeating Sequence Stair6/1 -> Sum6/2
  Repeating Sequence7/1 -> Sum7/1
  Repeating Sequence Stair7/1 -> Sum7/2
  Repeating Sequence8/1 -> Sum8/1
  Repeating Sequence Stair8/1 -> Sum8/2
  Repeating Sequence9/1 -> Sum9/1
  Repeating Sequence Stair9/1 -> Sum9/2
  Repeating Sequence Stair/1 -> Sum/2
  Sum6/1 -> Relational Operator6/1, Mux6/7
  Sum7/1 -> Mux6/8, Relational Operator7/1
  Sum8/1 -> Relational Operator8/1, Mux6/9
  Sum9/1 -> Mux6/10, Relational Operator9/1
  Mux6/1 -> Scope1/1
  connections:
  Full-Bridge Converter2/LConn2 -- Full-Bridge Converter3/LConn1
  +3/RConn1 -- Full-Bridge Converter2/RConn1
  -2/RConn1 -- Full-Bridge Converter1/RConn2
  Full-Bridge Converter1/LConn2 -- Full-Bridge Converter2/LConn1
  Full-Bridge Converter4/LConn2 -- Vout/RConn1
  +1/RConn1 -- Full-Bridge Converter/RConn1
  Full-Bridge Converter/LConn1 -- Vin/RConn1
  -4/RConn1 -- Full-Bridge Converter3/RConn2
  -1/RConn1 -- Full-Bridge Converter/RConn2
  +4/RConn1 -- Full-Bridge Converter3/RConn1
  -3/RConn1 -- Full-Bridge Converter2/RConn2
  Full-Bridge Converter4/LConn1 -- Full-Bridge Converter3/LConn2
  +5/RConn1 -- Full-Bridge Converter4/RConn1
  +2/RConn1 -- Full-Bridge Converter1/RConn1
  -5/RConn1 -- Full-Bridge Converter4/RConn2
  Full-Bridge Converter/LConn2 -- Full-Bridge Converter1/LConn1

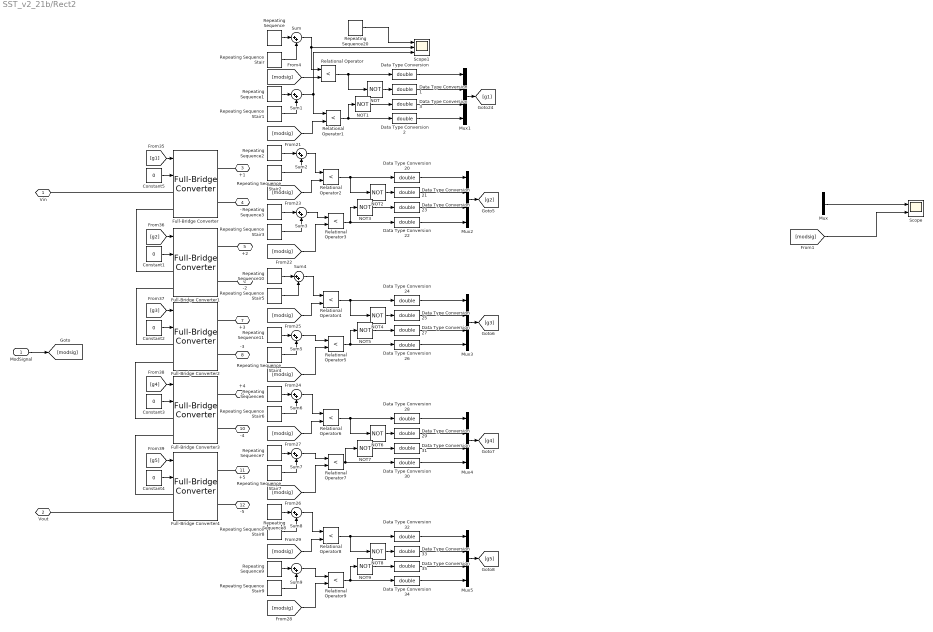
== system SST_v2_21b/Rect2 ==
  ModSignal : Inport
  Constant{1..5} (5 alike) : Constant  Value=0
  Data Type Conversion{,1..3,20..35} (20 alike) : DataTypeConversion  OutMin=[0]  OutMax=[1]  OutDataTypeStr=double
  Full-Bridge Converter{,1..4} (5 alike) : spsFullBridgeConverterLib/Full-Bridge Converter  ModelType=Switching devices  Ron=Rdson  Rs=Rsnubber  Cs=Csnubber  Vforward=[0,0]  Ron_Diode=1e-3  Rs_Diode=1e6  Cs_Diode=inf  Vf_Diode=1e-3  Rs_CurrentSource=inf
      settings: SourceProductBaseCode=PS
  Mux : Mux  Inputs=10
  Mux{1..5} (5 alike) : Mux
  NOT{,1..9} (10 alike) : Logic  Operator=NOT  IconShape=distinctive  AllPortsSameDT=off  OutDataTypeStr=boolean
  Relational Operator{,1..9} (10 alike) : RelationalOperator  Operator=<  OutDataTypeStr=boolean  RndMeth=Simplest
  Repeating Sequence : simulink/Sources/Repeating Sequence  rep_seq_t=Tcarriers  rep_seq_y=Ac11
  Repeating Sequence Stair : simulink/Sources/Repeating Sequence Stair  OutValues=Sc11  tsamp=TswS  OutMin=[]  OutMax=[]  OutDataTypeStr=double  OutputDataTypeScalingMode=double  OutDataType=fixdt(0,8)  ConRadixGroup=Best Precision: Vector-wise  OutScaling=2^-12
  Repeating Sequence Stair1 : simulink/Sources/Repeating Sequence Stair  OutValues=Sc12  tsamp=TswS  OutMin=[]  OutMax=[]  OutDataTypeStr=double  OutputDataTypeScalingMode=double  OutDataType=fixdt(0,8)  ConRadixGroup=Best Precision: Vector-wise  OutScaling=2^-12
  Repeating Sequence Stair2 : simulink/Sources/Repeating Sequence Stair  OutValues=Sc21  tsamp=TswS  OutMin=[]  OutMax=[]  OutDataTypeStr=double  OutputDataTypeScalingMode=double  OutDataType=fixdt(0,8)  ConRadixGroup=Best Precision: Vector-wise  OutScaling=2^-12
  Repeating Sequence Stair3 : simulink/Sources/Repeating Sequence Stair  OutValues=Sc22  tsamp=TswS  OutMin=[]  OutMax=[]  OutDataTypeStr=double  OutputDataTypeScalingMode=double  OutDataType=fixdt(0,8)  ConRadixGroup=Best Precision: Vector-wise  OutScaling=2^-12
  Repeating Sequence Stair4 : simulink/Sources/Repeating Sequence Stair  OutValues=Sc32  tsamp=TswS  OutMin=[]  OutMax=[]  OutDataTypeStr=double  OutputDataTypeScalingMode=double  OutDataType=fixdt(0,8)  ConRadixGroup=Best Precision: Vector-wise  OutScaling=2^-12
  Repeating Sequence Stair5 : simulink/Sources/Repeating Sequence Stair  OutValues=Sc31  tsamp=TswS  OutMin=[]  OutMax=[]  OutDataTypeStr=double  OutputDataTypeScalingMode=double  OutDataType=fixdt(0,8)  ConRadixGroup=Best Precision: Vector-wise  OutScaling=2^-12
  Repeating Sequence Stair6 : simulink/Sources/Repeating Sequence Stair  OutValues=Sc41  tsamp=TswS  OutMin=[]  OutMax=[]  OutDataTypeStr=double  OutputDataTypeScalingMode=double  OutDataType=fixdt(0,8)  ConRadixGroup=Best Precision: Vector-wise  OutScaling=2^-12
  Repeating Sequence Stair7 : simulink/Sources/Repeating Sequence Stair  OutValues=Sc42  tsamp=TswS  OutMin=[]  OutMax=[]  OutDataTypeStr=double  OutputDataTypeScalingMode=double  OutDataType=fixdt(0,8)  ConRadixGroup=Best Precision: Vector-wise  OutScaling=2^-12
  Repeating Sequence Stair8 : simulink/Sources/Repeating Sequence Stair  OutValues=Sc51  tsamp=TswS  OutMin=[]  OutMax=[]  OutDataTypeStr=double  OutputDataTypeScalingMode=double  OutDataType=fixdt(0,8)  ConRadixGroup=Best Precision: Vector-wise  OutScaling=2^-12
  Repeating Sequence Stair9 : simulink/Sources/Repeating Sequence Stair  OutValues=Sc52  tsamp=TswS  OutMin=[]  OutMax=[]  OutDataTypeStr=double  OutputDataTypeScalingMode=double  OutDataType=fixdt(0,8)  ConRadixGroup=Best Precision: Vector-wise  OutScaling=2^-12
  Repeating Sequence1 : simulink/Sources/Repeating Sequence  rep_seq_t=Tcarriers  rep_seq_y=AC12
  Repeating Sequence10 : simulink/Sources/Repeating Sequence  rep_seq_t=Tcarriers  rep_seq_y=Ac31
  Repeating Sequence11 : simulink/Sources/Repeating Sequence  rep_seq_t=Tcarriers  rep_seq_y=AC32
  Repeating Sequence2 : simulink/Sources/Repeating Sequence  rep_seq_t=Tcarriers  rep_seq_y=Ac21
  Repeating Sequence20 : simulink/Sources/Repeating Sequence  rep_seq_t=Tcarriers  rep_seq_y=Ac11
  Repeating Sequence3 : simulink/Sources/Repeating Sequence  rep_seq_t=Tcarriers  rep_seq_y=Ac22
  Repeating Sequence6 : simulink/Sources/Repeating Sequence  rep_seq_t=Tcarriers  rep_seq_y=Ac41
  Repeating Sequence7 : simulink/Sources/Repeating Sequence  rep_seq_t=Tcarriers  rep_seq_y=Ac42
  Repeating Sequence8 : simulink/Sources/Repeating Sequence  rep_seq_t=Tcarriers  rep_seq_y=Ac51
  Repeating Sequence9 : simulink/Sources/Repeating Sequence  rep_seq_t=Tcarriers  rep_seq_y=Ac52
  Scope : Scope  NumInputPorts=2
  Scope1 : Scope  NumInputPorts=3
  Sum{,1..9} (10 alike) : Sum  Inputs=|++
  Vin : PMIOPort  Side=Left
  Vout : PMIOPort  Port=2  Side=Left
  +1 : PMIOPort  Port=3  Side=Right
  -1 : PMIOPort  Port=4  Side=Right
  +2 : PMIOPort  Port=5  Side=Right
  -2 : PMIOPort  Port=6  Side=Right
  +3 : PMIOPort  Port=7  Side=Right
  -3 : PMIOPort  Port=8  Side=Right
  +4 : PMIOPort  Port=9  Side=Right
  -4 : PMIOPort  Port=10  Side=Right
  +5 : PMIOPort  Port=11  Side=Right
  -5 : PMIOPort  Port=12  Side=Right
  wires:
  Data Type Conversion/1 -> Mux1/1
  [modsig] -> Relational Operator7/2
  Data Type Conversion33/1 -> Mux5/2
  NOT2/1 -> Data Type Conversion21/1
  Data Type Conversion30/1 -> Mux4/4
  Constant5/1 -> Full-Bridge Converter/2
  Data Type Conversion31/1 -> Mux4/3
  Data Type Conversion23/1 -> Mux2/3
  [g4] -> Full-Bridge Converter3/1
  NOT8/1 -> Data Type Conversion33/1
  Constant4/1 -> Full-Bridge Converter4/2
  Data Type Conversion29/1 -> Mux4/2
  Data Type Conversion24/1 -> Mux3/1
  Data Type Conversion25/1 -> Mux3/2
  NOT7/1 -> Data Type Conversion31/1
  Mux5/1 -> [g5]
  [g1] -> Full-Bridge Converter/1
  NOT5/1 -> Data Type Conversion27/1
  NOT3/1 -> Data Type Conversion23/1
  Relational Operator8/1 -> Data Type Conversion32/1, NOT8/1
  Data Type Conversion26/1 -> Mux3/4
  [modsig] -> Relational Operator6/2
  Relational Operator3/1 -> Data Type Conversion22/1, NOT3/1
  Mux1/1 -> [g1]
  Constant2/1 -> Full-Bridge Converter2/2
  Data Type Conversion3/1 -> Mux1/3
  Mux4/1 -> [g4]
  Relational Operator5/1 -> Data Type Conversion26/1, NOT5/1
  Relational Operator1/1 -> Data Type Conversion2/1, NOT1/1
  Constant1/1 -> Full-Bridge Converter1/2
  [modsig] -> Relational Operator3/2
  Relational Operator/1 -> Data Type Conversion/1, NOT/1
  [g2] -> Full-Bridge Converter1/1
  Mux2/1 -> [g2]
  Relational Operator4/1 -> Data Type Conversion24/1, NOT4/1
  [modsig] -> Relational Operator/2
  [modsig] -> Relational Operator9/2
  Data Type Conversion32/1 -> Mux5/1
  NOT/1 -> Data Type Conversion1/1
  Data Type Conversion35/1 -> Mux5/3
  Relational Operator6/1 -> Data Type Conversion28/1, NOT6/1
  [modsig] -> Relational Operator1/2
  NOT6/1 -> Data Type Conversion29/1
  NOT1/1 -> Data Type Conversion3/1
  [modsig] -> Relational Operator5/2
  Data Type Conversion21/1 -> Mux2/2
  Data Type Conversion27/1 -> Mux3/3
  Relational Operator2/1 -> Data Type Conversion20/1, NOT2/1
  Mux3/1 -> [g3]
  Relational Operator7/1 -> Data Type Conversion30/1, NOT7/1
  Data Type Conversion34/1 -> Mux5/4
  [modsig] -> Relational Operator4/2
  NOT9/1 -> Data Type Conversion35/1
  [g3] -> Full-Bridge Converter2/1
  Data Type Conversion28/1 -> Mux4/1
  Data Type Conversion20/1 -> Mux2/1
  Repeating Sequence3/1 -> Sum3/1
  [modsig] -> Relational Operator2/2
  Relational Operator9/1 -> Data Type Conversion34/1, NOT9/1
  [modsig] -> Relational Operator8/2
  Constant3/1 -> Full-Bridge Converter3/2
  Data Type Conversion1/1 -> Mux1/2
  NOT4/1 -> Data Type Conversion25/1
  Data Type Conversion2/1 -> Mux1/4
  Data Type Conversion22/1 -> Mux2/4
  [g5] -> Full-Bridge Converter4/1
  ModSignal/1 -> [modsig]
  Mux/1 -> Scope/1
  [modsig] -> Scope/2
  Repeating Sequence/1 -> Sum/1
  Sum/1 -> Scope1/2, Relational Operator/1
  Repeating Sequence1/1 -> Sum1/1
  Repeating Sequence Stair1/1 -> Sum1/2
  Sum1/1 -> Scope1/3, Relational Operator1/1
  Repeating Sequence2/1 -> Sum2/1
  Repeating Sequence Stair2/1 -> Sum2/2
  Sum2/1 -> Relational Operator2/1
  Sum3/1 -> Relational Operator3/1
  Repeating Sequence Stair3/1 -> Sum3/2
  Repeating Sequence10/1 -> Sum4/1
  Repeating Sequence Stair5/1 -> Sum4/2
  Sum4/1 -> Relational Operator4/1
  Repeating Sequence11/1 -> Sum5/1
  Sum5/1 -> Relational Operator5/1
  Repeating Sequence Stair4/1 -> Sum5/2
  Repeating Sequence6/1 -> Sum6/1
  Repeating Sequence Stair6/1 -> Sum6/2
  Sum6/1 -> Relational Operator6/1
  Repeating Sequence7/1 -> Sum7/1
  Repeating Sequence Stair7/1 -> Sum7/2
  Sum7/1 -> Relational Operator7/1
  Repeating Sequence8/1 -> Sum8/1
  Sum8/1 -> Relational Operator8/1
  Repeating Sequence Stair8/1 -> Sum8/2
  Repeating Sequence9/1 -> Sum9/1
  Repeating Sequence Stair9/1 -> Sum9/2
  Sum9/1 -> Relational Operator9/1
  Repeating Sequence20/1 -> Scope1/1
  Repeating Sequence Stair/1 -> Sum/2
  connections:
  Full-Bridge Converter2/LConn2 -- Full-Bridge Converter3/LConn1
  +3/RConn1 -- Full-Bridge Converter2/RConn1
  -2/RConn1 -- Full-Bridge Converter1/RConn2
  Full-Bridge Converter1/LConn2 -- Full-Bridge Converter2/LConn1
  Full-Bridge Converter4/LConn2 -- Vout/RConn1
  +1/RConn1 -- Full-Bridge Converter/RConn1
  Full-Bridge Converter/LConn1 -- Vin/RConn1
  -4/RConn1 -- Full-Bridge Converter3/RConn2
  -1/RConn1 -- Full-Bridge Converter/RConn2
  +4/RConn1 -- Full-Bridge Converter3/RConn1
  -3/RConn1 -- Full-Bridge Converter2/RConn2
  Full-Bridge Converter4/LConn1 -- Full-Bridge Converter3/LConn2
  +5/RConn1 -- Full-Bridge Converter4/RConn1
  +2/RConn1 -- Full-Bridge Converter1/RConn1
  -5/RConn1 -- Full-Bridge Converter4/RConn2
  Full-Bridge Converter/LConn2 -- Full-Bridge Converter1/LConn1
